simulink model "LoopShaping"  (R2019a)
settings: Solver=VariableStepAuto  StartTime=0.0  StopTime=5  RelTol=1e-3
values from neighbouring files (symbols this model uses):
  C = k*C    [Berard_LoopShaping.m]    (also in Berard_Modelo_ControlEE.m = [1 0 0])
  R = 100*(s+10)/(s+1000)    [Berard_LoopShaping.m]
libraries: cstblocks x2
settings Model: Creator=Duby  LastModifiedBy=ARLUBER1
settings DataIOCC: ReturnWorkspaceOutputs=off
settings DebuggingCC: ArithmeticOperatorsInVariantConditions=warning
settings SFSimCC: SimUseLocalCustomCode=off
settings RTWCC: RTWUseLocalCustomCode=off
settings CodeAppCC: StateflowObjectComments=on

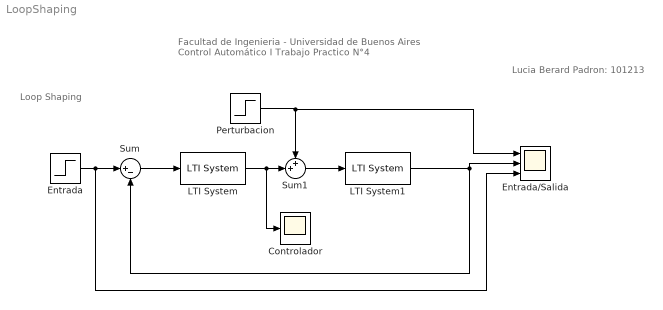
== system LoopShaping ==
  note: Loop Shaping
  note: Lucia Berard
      | Padron: 101213
  note: Facultad de Ingenieria - Universidad de Buenos Aires
      | Control Automático I
      | Trabajo Practico N°4
  Controlador : Scope
  Entrada : Step  SampleTime=0.001
  Entrada/Salida : Scope  NumInputPorts=3
  "LTI System " : cstblocks/LTI System  sys=R*C  IC=[]
  "LTI System1 " : cstblocks/LTI System  sys=H  IC=[]
  Perturbacion : Step  Time=3  After=1.2  SampleTime=0.001
  Sum : Sum  Inputs=|+-
  Sum1 : Sum  Inputs=++|
  wires:
  "LTI System1 "/1 -> Sum/2, Entrada/Salida/2
  Sum/1 -> "LTI System "/1
  Sum1/1 -> "LTI System1 "/1
  "LTI System "/1 -> Controlador/1, Sum1/2
  Entrada/1 -> Entrada/Salida/3, Sum/1
  Perturbacion/1 -> Entrada/Salida/1, Sum1/1
